simulink library "DoorRatSts"  (R2022a)
settings: Solver=VariableStepAuto  StartTime=0.0  StopTime=10.0  RelTol=1e-3
settings Model: Creator=DELL  LastModifiedBy=DELL

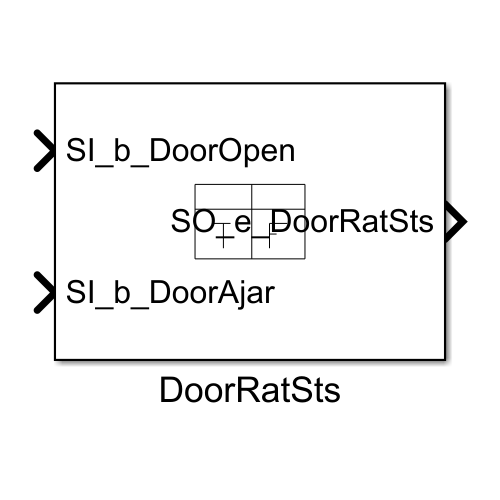
[thumbnail: Simulink's stored preview of the top-level diagram]
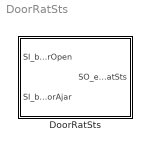
== system DoorRatSts ==
  DoorRatSts : Truth Table  TreatAsAtomicUnit=on

== matlab function DoorRatSts/DoorRatSts ==
  data: SI_b_DoorOpen input boolean; SO_e_DoorRatSts output Enum: DoorRat_Sts_E; SI_b_DoorAjar input boolean
function SO_e_DoorRatSts = fcn(SI_b_DoorOpen, SI_b_DoorAjar)

aVarTruthTableCondition_1 = false;
aVarTruthTableCondition_2 = false;


% condition 1

aVarTruthTableCondition_1 = logical(SI_b_DoorOpen == 1);

% condition 2

aVarTruthTableCondition_2 = logical(SI_b_DoorAjar == 1);

if (~aVarTruthTableCondition_1 && ~aVarTruthTableCondition_2)
    aFcnTruthTableAction_2();
elseif (~aVarTruthTableCondition_1 && aVarTruthTableCondition_2)
    aFcnTruthTableAction_3();
elseif (aVarTruthTableCondition_1 && aVarTruthTableCondition_2)
    aFcnTruthTableAction_4();
else % Default
    aFcnTruthTableAction_1();
end

function aFcnTruthTableAction_1()

% Invalid

SO_e_DoorRatSts = Invalid;

function aFcnTruthTableAction_2()

% All Lock

SO_e_DoorRatSts = All_Lock;

function aFcnTruthTableAction_3()

% Half Lock

SO_e_DoorRatSts = Half_Lock;

function aFcnTruthTableAction_4()

% Unlock

SO_e_DoorRatSts = Unlock;
